simulink model "DWorkAnalysisJonasSpesial"  (R2021b)
settings: Solver=FixedStepAuto  StartTime=0.0  StopTime=60  FixedStep=0.1  RelTol=1e-3
model workspace (MATLAB code in the model file):
  | %% Mechanical Parameters
  | d_Drum = 23.23e-2; % Meter
  | Drum_Friction = 0.001; % Ns/m
  | Drum_Inertia = 1.0; %kgm^2
  | 
  | n_sh = 5;
  | 
  | %% Load Case 1
  | Hs = 2.2; % m
  | T_w = 8.0; % s
  | m_payload = 8000; % kg
  | h_payload_0 = 75; % m
  | h_payload_final = h_payload_0; % m
  | h_seabed = 350; % m
  | 
  | %% Load Case 2
  | Hs = 2.2; % m
  | T_w = 8.0; % s
  | m_payload = 8000; % kg
  | h_payload_0 = 75; % m
  | h_payload_final = 15; % m
  | h_seabed = 350; % m
  | 
  | %% Load Case 3
  | Hs = 2.2; % m
  | T_w = 8.0; % s
  | m_payload = 8000; % kg
  | h_payload_0 =15; % m
  | h_payload_final = 0; % m
  | h_seabed = 350; % m
  | 
  | %% Sensors
  | % Noise simulation
  | sigma_w = 0.5; %m/s^2 (Standard deviation of noise)
  | beta = 10000; % Positive constant [-]
  | 
  | %% Payload parameters
  | % mass already defined (8000kg)
  | Volume_pl = 2; %m^3
  | Area_pl = 1.5; %m^2
  | C_D = 1.8; %[-] Drag coefficient
  | 
  | %syms rho vel
  | %F_drag = 0.5 * rho * vel^2 * C_D * Area_pl; % Density of sea water(surface) approx 1.025 kg/m^3, velocity comes from the simulation.
  | 
  | %% Seabed
  | k_spring = 1.8e6; %N/m
  | b_damper = 6.5e5; %Ns/m
  | rho = 1.025;
  | %syms delta_x
  | %if delta_x < 0
  | %    F_sb = 0;
  | %else
  | %    F_sb = k_spring*delta_x + b_damper*vel*sqrt(delta_x);
  | %end
  | 
  | %% Bouyant force
  | % The force pushing upwards when something floats down in water. Dependend
  | % on the fluid density, volume of the object falling and gravity
  | g = 9.81;
  | %F_boy = rho * Volume_pl * g;
libraries: fl_lib x20, nesl_utility x8, CustomComponents_lib x6, slpidlib x1, simulink x1
settings Model: Creator=Jakob  LastModifiedBy=katri
settings DebuggingCC: AlgebraicLoopMsg=none  UnconnectedInputMsg=none  UnconnectedOutputMsg=none  UnconnectedLineMsg=none
settings RTWCC: DLArmComputeVersion=20.02.1

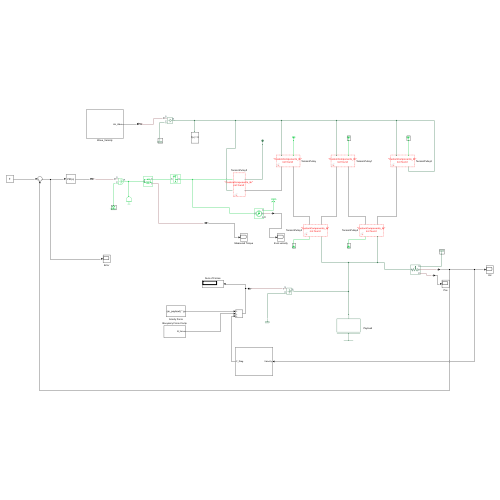
[thumbnail: Simulink's stored preview of the top-level diagram]
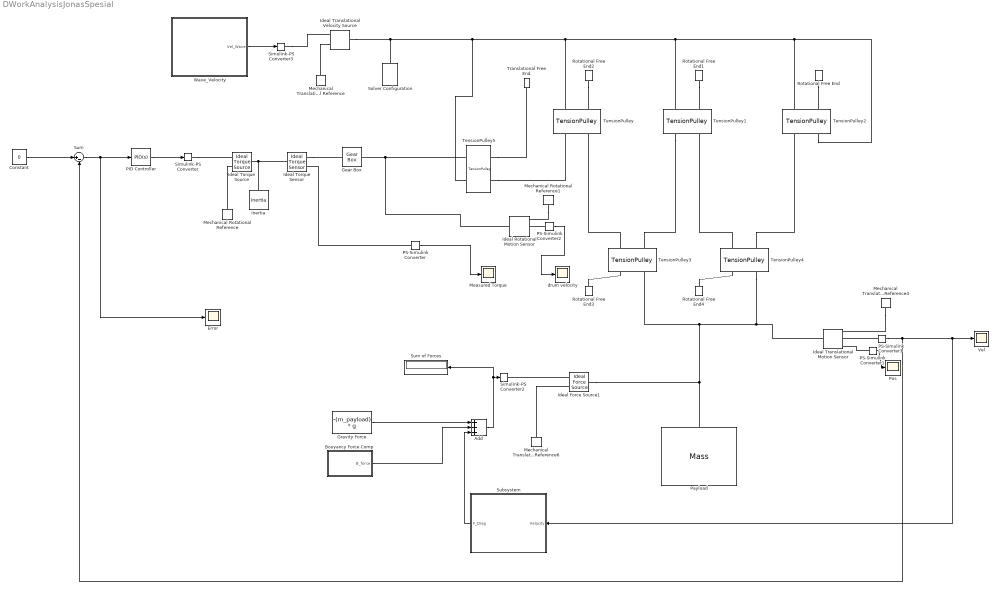
== system DWorkAnalysisJonasSpesial ==
  Add : Sum  Inputs=+++
  Bouyancy Force Comp : Subsystem
  Constant : Constant  Value=0
  Error : Scope
  Gear Box : fl_lib/Mechanical/Mechanisms/Gear Box  ratio=6  t_in_specify=off  t_in_priority=None  t_in=0 N*m  t_in_nominal_specify=off  t_in_nominal_unit=N*m  t_in_nominal_value=1  t_out_specify=off  t_out_priority=None  t_out=0 N*m  t_out_nominal_specify=off  t_out_nominal_unit=N*m  t_out_nominal_value=1
  Gravity Force : Constant  Value=-(m_payload) * g
  Ideal Force Source1 : fl_lib/Mechanical/Mechanical Sources/Ideal Force Source
  Ideal Rotational Motion Sensor : fl_lib/Mechanical/Mechanical Sensors/Ideal Rotational Motion Sensor  reference=foundation.enum.MeasurementReference.difference  acceleration_port=false  velocity_port=true  position_port=true  wrap_angle=simscape.enum.onoff.off  offset=0 rad
  Ideal Torque Sensor : fl_lib/Mechanical/Mechanical Sensors/Ideal Torque Sensor
  Ideal Torque Source : fl_lib/Mechanical/Mechanical Sources/Ideal Torque Source
  Ideal Translational Motion Sensor : fl_lib/Mechanical/Mechanical Sensors/Ideal Translational Motion Sensor  reference=foundation.enum.MeasurementReference.difference  acceleration_port=false  velocity_port=true  position_port=true  offset=75 m
  Ideal Translational Velocity Source : fl_lib/Mechanical/Mechanical Sources/Ideal Translational Velocity Source
  Inertia : fl_lib/Mechanical/Rotational Elements/Inertia  inertia=3.4 kg*m^2  num_ports=foundation.enum.numPorts2.one  w_specify=off  w_priority=High  w=0 rad/s  w_nominal_specify=off  w_nominal_unit=rad/s  w_nominal_value=1  t_specify=off  t_priority=None  t=0 N*m  t_nominal_specify=off  t_nominal_unit=N*m  t_nominal_value=1
  Measured Torque : Scope
  Mechanical Rotational Reference : fl_lib/Mechanical/Rotational Elements/Mechanical Rotational Reference
  Mechanical Rotational Reference1 : fl_lib/Mechanical/Rotational Elements/Mechanical Rotational Reference
  Mechanical Translational Reference : fl_lib/Mechanical/Translational Elements/Mechanical Translational Reference
  Mechanical Translational Reference4 : fl_lib/Mechanical/Translational Elements/Mechanical Translational Reference
  Mechanical Translational Reference6 : fl_lib/Mechanical/Translational Elements/Mechanical Translational Reference
  PID Controller : slpidlib/PID Controller  Controller=PID  Form=Parallel  TimeDomain=Continuous-time  UseExternalTs=off  SampleTime=-1  IntegratorMethod=Forward Euler  FilterMethod=Forward Euler  ControllerParametersSource=internal  P=2000  I=500  D=250  N=100  UseFilter=on  TunerSelectOption=Transfer Function Based (PID Tuner App)  InitialConditionSource=internal  InitialConditionForIntegrator=0  InitialConditionForFilter=0  DifferentiatorICPrevScaledInput=0  ExternalReset=none  TrackingMode=off  Kt=1  LimitOutput=off  SatLimitsSource=internal  UpperSaturationLimit=inf  LowerSaturationLimit=-inf  LinearizeAsGain=on  AntiWindupMode=none  Kb=1  POutMin=[]  POutMax=[]  IOutMin=[]  IOutMax=[]  DOutMin=[]  DOutMax=[]  NOutMin=[]  NOutMax=[]  SumOutMin=[]  SumOutMax=[]  SaturationOutMin=[]  SaturationOutMax=[]  PParamMin=[]  PParamMax=[]  IParamMin=[]  IParamMax=[]  DParamMin=[]  DParamMax=[]  NParamMin=[]  NParamMax=[]  KbParamMin=[]  KbParamMax=[]  KtParamMin=[]  KtParamMax=[]  KbOutMin=[]  KbOutMax=[]  KtOutMin=[]  KtOutMax=[]  IntegratorOutMin=[]  IntegratorOutMax=[]  FilterOutMin=[]  FilterOutMax=[]  SumI1OutMin=[]  SumI1OutMax=[]  SumI2OutMin=[]  SumI2OutMax=[]  SumI3OutMin=[]  SumI3OutMax=[]  SumI4OutMin=[]  SumI4OutMax=[]  SumDOutMin=[]  SumDOutMax=[]  DifferentiatorOutMin=[]  DifferentiatorOutMax=[]  FilterDiffOutCoefMin=[]  FilterDiffOutCoefMax=[]  ReciprocalOutMin=[]  ReciprocalOutMax=[]  SumDenOutMin=[]  SumDenOutMax=[]  SumNumOutMin=[]  SumNumOutMax=[]  DivideOutMin=[]  DivideOutMax=[]  UdiffTsProdOutMin=[]  UdiffTsProdOutMax=[]  NTsProdOutMin=[]  NTsProdOutMax=[]  UintegralTsProdOutMin=[]  UintegralTsProdOutMax=[]  UngainTsProdOutMin=[]  UngainTsProdOutMax=[]  IntegratorContinuousStateAttributes=''  IntegratorStateMustResolveToSignalObject=off  IntegratorRTWStateStorageClass=Auto  FilterContinuousStateAttributes=''  FilterStateMustResolveToSignalObject=off  FilterRTWStateStorageClass=Auto  ParallelPVariant=InternalParameters  IdealPVariant=Disabled  IVariant=InternalParameters  DVariant=InternalParameters  IntegratorVariant=Continuous  SatVariant=Disabled  AWVariant=Passthrough  PCopyVariant=Disabled  TRVariant=Disabled  FdbkBlocksVariant=Forward  IdealPFdbkVariant=Disabled  SatFdbkVariant=Disabled  DerivativeFilterVariant=ContFilter  NVariant=InternalParameters  NCopyVariant=Disabled  FilterICVariant=InternalICsFilter  IntegratorICVariant=InternalICs  ExternalResetVariant=Disabled  TRSumVariant=Passthrough  SumFdbkVariant=Disabled  SumVariant=Sum_PID  TsampFilterVariant=InternalTs  TsampNgainVariant=Passthrough  TsampIntegralVariant=Passthrough  ExternalSaturationOutDataTypeStr=Inherit: Same as second input
  PS-Simulink Converter{,1..3} (4 alike) : nesl_utility/PS-Simulink Converter  PhysicalDomain=network_engine_domain  SubClassName=ps_output  LeftPortType=input  RightPortType=output  PseudoPeriodic=off  Frequencies=[]  VectorFormat=inherit  Unit=inherit  AffineConversion=off
  Payload : fl_lib/Mechanical/Translational Elements/Mass  mass=0.01 kg  num_ports=foundation.enum.numPorts2.one  v_specify=off  v_priority=High  v=0 m/s  v_nominal_specify=off  v_nominal_unit=m/s  v_nominal_value=1  f_specify=off  f_priority=None  f=0 N  f_nominal_specify=off  f_nominal_unit=N  f_nominal_value=1
  Pos : Scope
  Rotational Free End{,1..4} (5 alike) : fl_lib/Mechanical/Rotational Elements/Rotational Free End  w_specify=off  w_priority=None  w=0 rad/s  w_nominal_specify=off  w_nominal_unit=rad/s  w_nominal_value=1
  Simulink-PS Converter : nesl_utility/Simulink-PS Converter  PhysicalDomain=network_engine_domain  SubClassName=ps_input  LeftPortType=input  RightPortType=output  PseudoPeriodic=off  Frequencies=[]  NoiseDistribution=none  NoiseParameters=[]  Unit=1  AffineConversion=off  FilteringAndDerivatives=provide  SimscapeFilterOrder=1  InputFilterTimeConstant=0.001  UdotUserProvided=0
  Simulink-PS Converter2 : nesl_utility/Simulink-PS Converter  PhysicalDomain=network_engine_domain  SubClassName=ps_input  LeftPortType=input  RightPortType=output  PseudoPeriodic=off  Frequencies=[]  NoiseDistribution=none  NoiseParameters=[]  Unit=1  AffineConversion=off  FilteringAndDerivatives=provide  SimscapeFilterOrder=1  InputFilterTimeConstant=0.001  UdotUserProvided=0
  Simulink-PS Converter3 : nesl_utility/Simulink-PS Converter  PhysicalDomain=network_engine_domain  SubClassName=ps_input  LeftPortType=input  RightPortType=output  PseudoPeriodic=off  Frequencies=[]  NoiseDistribution=none  NoiseParameters=[]  Unit=1  AffineConversion=off  FilteringAndDerivatives=filter  SimscapeFilterOrder=2  InputFilterTimeConstant=0.001  UdotUserProvided=0
  Solver Configuration : nesl_utility/Solver Configuration  PhysicalDomain=network_engine_domain  SubClassName=solver  LeftPortType=input  RightPortType=generic  Tones=[]  Harmonics=[]  SimulateNoise=off  Profile=off  UseLocalSampling=off  EnableSwitchedLinearOptims=on  FrequencyDomain=off  UseCCode=off  RelTol=0.001  AbsTol=0.001  MinStep=1e-09  ToWorkspace=off  RevertToSquareIcSolve=off  NumHomotopyIterations=100  PhasorMode=off  PhasorModeNumHarmonics=1  ConsistencySolver=NEWTON_FTOL  IndexReductionMethod=DerivativeReplacement  DoDC=off  ResidualTolerance=1e-09  ConsistencyTolSource=GLOBAL  ConsistencyAbsTol=0.001  ConsistencyRelTol=0.001  ConsistencyTolFactor=0.001  UseLocalSolver=off  LocalSolverChoice=NE_BACKWARD_EULER_ADVANCER  ResolveIndetEquations=on  FunctionEvalNumThread=1  LocalSolverSampleTime=0.001  DoFixedCost=off  MaxNonlinIter=3  MaxModeIter=2  ComputeImpulses=off  ImpulseIterations=2  LinearAlgebra=auto  LinearAlgebraNumThread=0  EquationFormulation=NE_TIME_EF  DelaysMemoryBudget=1024  AutomaticFiltering=on  FilteringTimeConstant=0.001  PartitionStorageMethod=AS_NEEDED  PartitionMemoryBudget=1024  PartitionMethod=ROBUST
  Subsystem : Subsystem
  Sum : Sum  Inputs=|+-
  Sum of Forces : Display
  TensionPulley{,1..2,4} (4 alike) : CustomComponents_lib/TensionPulley  radius=0.1 m  b_damp=0 N*m*s/rad  inertia=0.00001 kg*m^2  mass=0.1 kg  mu_s=1  f_A_specify=off  f_A_priority=None  f_A=0 N  f_A_nominal_specify=off  f_A_nominal_unit=N  f_A_nominal_value=1  f_B_specify=off  f_B_priority=None  f_B=0 N  f_B_nominal_specify=off  f_B_nominal_unit=N  f_B_nominal_value=1  f_C_specify=off  f_C_priority=None  f_C=0 N  f_C_nominal_specify=off  f_C_nominal_unit=N  f_C_nominal_value=1  tau_specify=off  tau_priority=None  tau=0 N*m  tau_nominal_specify=off  tau_nominal_unit=N*m  tau_nominal_value=1  w_specify=off  w_priority=None  w=0 rad/s  w_nominal_specify=off  w_nominal_unit=rad/s  w_nominal_value=1  v_specify=off  v_priority=None  v=0 m/s  v_nominal_specify=off  v_nominal_unit=m/s  v_nominal_value=1
      settings: InternalSimscapePortConfiguration="{\"Bottom\":[],\"Left\":[{\"id\":\"C\",\"label\":\"C\",\"type\":\"foundation.mechanical.translational.translational\"},{\"id\":\"S\",\"label\":\"S\",\"type\":\"foundation.mechanical.rotational.rotational\"}],\"Right\":[{\"id\":\"A\",\"label\":\"A\",\"type\":\"foundation.mechanical.translational.translational\"},{\"id\":\"B\",\"label\":\"B\",\"type\":\"foundation.mechanical.translational.translational\"}],\"Top\":[]}"
  TensionPulley3 : CustomComponents_lib/TensionPulley  radius=0.1 m  b_damp=0 N*m*s/rad  inertia=00.00001 kg*m^2  mass=0.1 kg  mu_s=1  f_A_specify=off  f_A_priority=None  f_A=0 N  f_A_nominal_specify=off  f_A_nominal_unit=N  f_A_nominal_value=1  f_B_specify=off  f_B_priority=None  f_B=0 N  f_B_nominal_specify=off  f_B_nominal_unit=N  f_B_nominal_value=1  f_C_specify=off  f_C_priority=None  f_C=0 N  f_C_nominal_specify=off  f_C_nominal_unit=N  f_C_nominal_value=1  tau_specify=off  tau_priority=None  tau=0 N*m  tau_nominal_specify=off  tau_nominal_unit=N*m  tau_nominal_value=1  w_specify=off  w_priority=None  w=0 rad/s  w_nominal_specify=off  w_nominal_unit=rad/s  w_nominal_value=1  v_specify=off  v_priority=None  v=0 m/s  v_nominal_specify=off  v_nominal_unit=m/s  v_nominal_value=1
      settings: InternalSimscapePortConfiguration="{\"Bottom\":[],\"Left\":[{\"id\":\"C\",\"label\":\"C\",\"type\":\"foundation.mechanical.translational.translational\"},{\"id\":\"S\",\"label\":\"S\",\"type\":\"foundation.mechanical.rotational.rotational\"}],\"Right\":[{\"id\":\"A\",\"label\":\"A\",\"type\":\"foundation.mechanical.translational.translational\"},{\"id\":\"B\",\"label\":\"B\",\"type\":\"foundation.mechanical.translational.translational\"}],\"Top\":[]}"
  TensionPulley5 : CustomComponents_lib/TensionPulley  radius=d_Drum m  b_damp=Drum_Friction N*m*s/rad  inertia=Drum_Inertia kg*m^2  mass=0.1 kg  mu_s=1  f_A_specify=off  f_A_priority=None  f_A=0 N  f_A_nominal_specify=off  f_A_nominal_unit=N  f_A_nominal_value=1  f_B_specify=off  f_B_priority=None  f_B=0 N  f_B_nominal_specify=off  f_B_nominal_unit=N  f_B_nominal_value=1  f_C_specify=off  f_C_priority=None  f_C=0 N  f_C_nominal_specify=off  f_C_nominal_unit=N  f_C_nominal_value=1  tau_specify=off  tau_priority=None  tau=0 N*m  tau_nominal_specify=off  tau_nominal_unit=N*m  tau_nominal_value=1  w_specify=off  w_priority=None  w=0 rad/s  w_nominal_specify=off  w_nominal_unit=rad/s  w_nominal_value=1  v_specify=off  v_priority=None  v=0 m/s  v_nominal_specify=off  v_nominal_unit=m/s  v_nominal_value=1
      settings: InternalSimscapePortConfiguration="{\"Bottom\":[],\"Left\":[{\"id\":\"C\",\"label\":\"C\",\"type\":\"foundation.mechanical.translational.translational\"},{\"id\":\"S\",\"label\":\"S\",\"type\":\"foundation.mechanical.rotational.rotational\"}],\"Right\":[{\"id\":\"A\",\"label\":\"A\",\"type\":\"foundation.mechanical.translational.translational\"},{\"id\":\"B\",\"label\":\"B\",\"type\":\"foundation.mechanical.translational.translational\"}],\"Top\":[]}"
  Translational Free End : fl_lib/Mechanical/Translational Elements/Translational Free End  v_specify=off  v_priority=None  v=0 m/s  v_nominal_specify=off  v_nominal_unit=m/s  v_nominal_value=1
      settings: InternalSimscapePortConfiguration="{\"Bottom\":[],\"Left\":[{\"id\":\"V\",\"label\":\"\",\"type\":\"foundation.mechanical.translational.translational\"}],\"Right\":[],\"Top\":[]}"
  Vel : Scope
  Wave_Velocity : Subsystem
  drum velocity : Scope
  wires:
  PS-Simulink Converter/1 -> Measured Torque/1
  PS-Simulink Converter1/1 -> Pos/1
  PS-Simulink Converter2/1 -> drum velocity/1
  PS-Simulink Converter3/1 -> Subsystem/1(Velocity), Vel/1, Sum/2
  Sum/1 -> PID Controller/1, Error/1
  PID Controller/1 -> Simulink-PS Converter/1
  Wave_Velocity/1(Vel_Wave) -> Simulink-PS Converter3/1
  Bouyancy Force Comp/1(B_force) -> Add/2
  Gravity Force/1 -> Add/1
  Add/1 -> Sum of Forces/1, Simulink-PS Converter2/1
  Subsystem/1(F_Drag) -> Add/3
  Constant/1 -> Sum/1
  connections:
  TensionPulley3/RConn2 -- TensionPulley/RConn2
  TensionPulley1/RConn1 -- TensionPulley3/RConn1
  TensionPulley4/RConn2 -- TensionPulley1/RConn2
  TensionPulley4/RConn1 -- TensionPulley2/RConn1
  Rotational Free End/LConn1 -- TensionPulley2/LConn2
  Rotational Free End1/LConn1 -- TensionPulley1/LConn2
  Rotational Free End2/LConn1 -- TensionPulley/LConn2
  Solver Configuration/RConn1 -- Ideal Translational Velocity Source/LConn1 -- TensionPulley5/LConn1 -- TensionPulley2/LConn1 -- TensionPulley2/RConn2 -- TensionPulley1/LConn1 -- TensionPulley/LConn1
  Rotational Free End3/LConn1 -- TensionPulley3/LConn2
  Rotational Free End4/LConn1 -- TensionPulley4/LConn2
  TensionPulley4/LConn1 -- Ideal Translational Motion Sensor/LConn1 -- Payload/LConn1 -- Ideal Force Source1/LConn1 -- TensionPulley3/LConn1
  Ideal Torque Sensor/RConn1 -- Gear Box/LConn1
  PS-Simulink Converter/LConn1 -- Ideal Torque Sensor/RConn2
  Simulink-PS Converter/RConn1 -- Ideal Torque Source/RConn1
  Ideal Torque Source/LConn1 -- Inertia/LConn1 -- Ideal Torque Sensor/LConn1
  Mechanical Rotational Reference/LConn1 -- Ideal Torque Source/RConn2
  PS-Simulink Converter1/LConn1 -- Ideal Translational Motion Sensor/RConn3
  Mechanical Translational Reference4/LConn1 -- Ideal Translational Motion Sensor/RConn1
  PS-Simulink Converter2/LConn1 -- Ideal Rotational Motion Sensor/RConn2
  Mechanical Rotational Reference1/LConn1 -- Ideal Rotational Motion Sensor/RConn1
  Ideal Rotational Motion Sensor/LConn1 -- TensionPulley5/LConn2 -- Gear Box/RConn1
  Ideal Force Source1/RConn1 -- Simulink-PS Converter2/RConn1
  Mechanical Translational Reference6/LConn1 -- Ideal Force Source1/RConn2
  PS-Simulink Converter3/LConn1 -- Ideal Translational Motion Sensor/RConn2
  Simulink-PS Converter3/RConn1 -- Ideal Translational Velocity Source/RConn1
  Mechanical Translational Reference/LConn1 -- Ideal Translational Velocity Source/RConn2
  TensionPulley5/RConn1 -- TensionPulley/RConn1
  TensionPulley5/RConn2 -- Translational Free End/LConn1

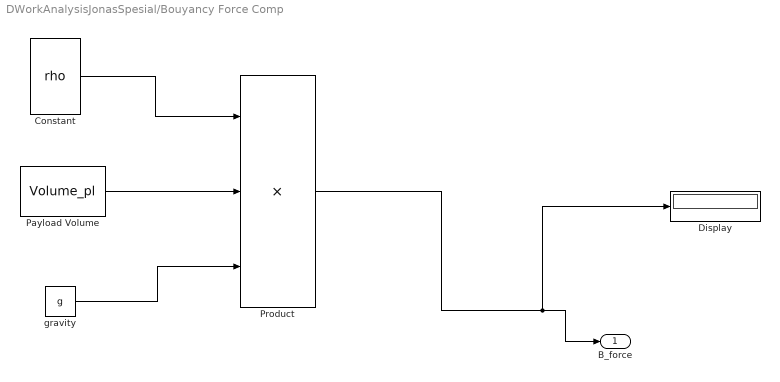
== system DWorkAnalysisJonasSpesial/Bouyancy Force Comp ==
  Constant : Constant  Value=rho
  Display : Display
  Payload Volume : Constant  Value=Volume_pl
  Product : Product  Inputs=3
  gravity : Constant  Value=g
  B_force : Outport
  wires:
  Constant/1 -> Product/1
  Payload Volume/1 -> Product/2
  gravity/1 -> Product/3
  Product/1 -> Display/1, B_force/1

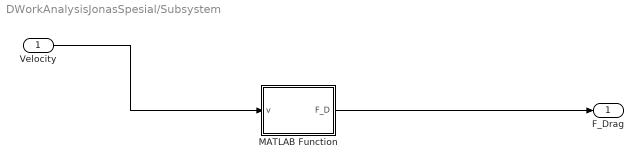
== system DWorkAnalysisJonasSpesial/Subsystem ==
  Velocity : Inport
  MATLAB Function : MATLAB Function  TreatAsAtomicUnit=on
  F_Drag : Outport
  wires:
  Velocity/1 -> MATLAB Function/1(v)
  MATLAB Function/1(F_D) -> F_Drag/1

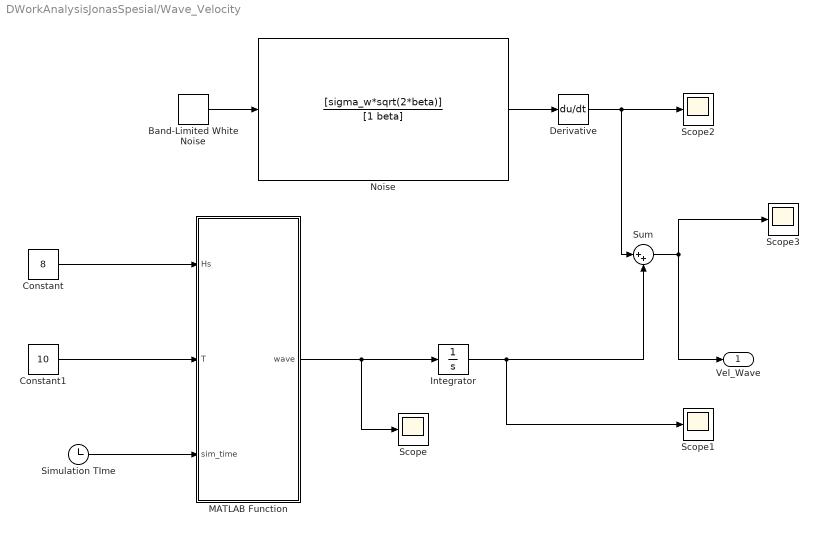
== system DWorkAnalysisJonasSpesial/Wave_Velocity ==
  Band-Limited White Noise : simulink/Sources/Band-Limited White Noise  Cov=[1]  Ts=0.1  seed=[23341]
  Constant : Constant  Value=8
  Constant1 : Constant  Value=10
  Derivative : Derivative
  Integrator : Integrator
  MATLAB Function : MATLAB Function  TreatAsAtomicUnit=on
  Noise : TransferFcn  Numerator=[sigma_w*sqrt(2*beta)]  Denominator=[1 beta]
  Scope{,1..3} (4 alike) : Scope
  Simulation TIme : Clock
      settings: Decimation=100
  Sum : Sum  Inputs=|++
  Vel_Wave : Outport
  wires:
  Constant/1 -> MATLAB Function/1(Hs)
  Simulation TIme/1 -> MATLAB Function/3(sim_time)
  MATLAB Function/1(wave) -> Integrator/1, Scope/1
  Constant1/1 -> MATLAB Function/2(T)
  Integrator/1 -> Sum/2, Scope1/1
  Noise/1 -> Derivative/1
  Band-Limited White Noise/1 -> Noise/1
  Derivative/1 -> Sum/1, Scope2/1
  Sum/1 -> Scope3/1, Vel_Wave/1

== matlab function DWorkAnalysisJonasSpesial/Wave_Velocity/MATLAB Function ==
  settings: updateMethod=DISCRETE
  data: Hs input; T input; sim_time input; wave output
function wave  = fcn(Hs, T, sim_time)
%WAVE GEN generates stochastic waves
% Hs is the significant wave height [m]
% T is the mean period [s]
% t end is the end time [s]
% t is the time [s]
% wave is sea surface elevation [m]
%% Input parameters
w = linspace (0.1, 2.0, 20); % frequency range
delta_w = w(2) - w(1);
%% PM spectrum (freq. domain )
w1 = (2*pi)/T;
A = 0.11*(Hs^2)*(w1^4);
B = 0.44*(w1^4);
S = (A./w.^5).* exp(-(B./w.^4));
%% Wave amplitude (time domain)
%sfr = 1/25 ; % sampling frequency (Hz) (higher freq −> higher resolution)
t = sim_time; % time vector
phi_test = rng;
phi = 2*pi*(rand(1,length (w))-0.5); % random phase of ith frequency [rad]
rng(phi_test);
A_wave = sqrt(2*S.*delta_w); % amplitude of each sine wave. wave = [] ;

wave = [sum(A_wave .*cos(w.*t + phi))]; % [m] sea surface elevation

== matlab function DWorkAnalysisJonasSpesial/Subsystem/MATLAB Function ==
  data: v input; F_D output
function F_D = fcn(v)
rho = 1.025;
C_D = 1.8;
Area_pl = 1.5; 


F_D = 0.5*rho*v^2*C_D*Area_pl;
